simulink model "fullmodel"  (R2024b)
settings: Solver=VariableStepAuto  StartTime=0.0  StopTime=10.0  RelTol=1e-3
libraries: simulink x1
settings Model: Creator=ryandavis  LastModifiedBy=Cory

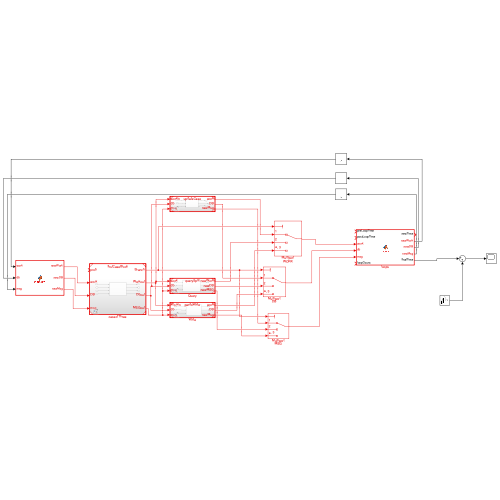
[thumbnail: Simulink's stored preview of the top-level diagram]
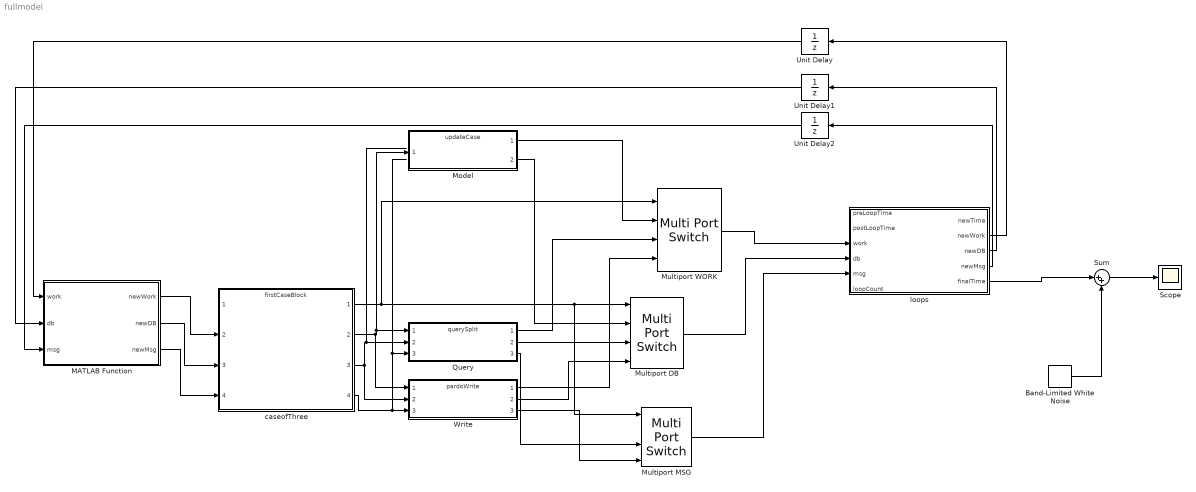
== system fullmodel ==
  Band-Limited White Noise : simulink/Sources/Band-Limited White Noise  Cov=[0.1]  Ts=0.1  seed=[23341]
  MATLAB Function : MATLAB Function  TreatAsAtomicUnit=on
  Model : ModelReference  ModelNameDialog=updateCase.slx  SimulationMode=Normal  ModelReferenceVersion=1.5
  Multiport DB : MultiPortSwitch  SaturateOnIntegerOverflow=off  InputSameDT=off
  Multiport MSG : MultiPortSwitch  SaturateOnIntegerOverflow=off  InputSameDT=off
  Multiport WORK : MultiPortSwitch  SaturateOnIntegerOverflow=off  InputSameDT=off
  Query : ModelReference  ModelNameDialog=querySplit.slx  SimulationMode=Normal  ModelReferenceVersion=1.7
  Scope : Scope
  Sum : Sum  Inputs=|++
  Unit Delay : UnitDelay  SampleTime=-1  HasFrameUpgradeWarning=on
  Unit Delay1 : UnitDelay  SampleTime=-1  HasFrameUpgradeWarning=on
  Unit Delay2 : UnitDelay  SampleTime=-1  HasFrameUpgradeWarning=on
  Write : ModelReference  ModelNameDialog=pardoWrite.slx  SimulationMode=Normal  ModelReferenceVersion=1.7
  caseofThree : ModelReference  ModelNameDialog=firstCaseBlock.slx  SimulationMode=Normal  ModelReferenceVersion=1.5
  loops : MATLAB Function  TreatAsAtomicUnit=on
  wires:
  MATLAB Function/3(newMsg) -> caseofThree/4
  MATLAB Function/2(newDB) -> caseofThree/3
  MATLAB Function/1(newWork) -> caseofThree/2
  caseofThree/1 -> Multiport WORK/1, Multiport MSG/1, Multiport DB/1
  Model/1 -> Multiport WORK/2
  Query/1 -> Multiport WORK/3
  Write/1 -> Multiport WORK/4
  Model/2 -> Multiport DB/2
  Query/2 -> Multiport DB/3
  ? -> Multiport MSG/2
  Write/2 -> Multiport DB/4
  Query/3 -> Multiport MSG/3
  Write/3 -> Multiport MSG/4
  Multiport WORK/1 -> loops/3(work)
  Multiport DB/1 -> loops/4(db)
  Multiport MSG/1 -> loops/5(msg)
  caseofThree/2 -> Write/1, Query/1, Model/1
  caseofThree/3 -> Write/2, Query/2
  caseofThree/4 -> Query/3, Write/3
  loops/5(finalTime) -> Sum/1
  Band-Limited White Noise/1 -> Sum/2
  Sum/1 -> Scope/1
  loops/2(newWork) -> Unit Delay/1
  loops/3(newDB) -> Unit Delay1/1
  loops/4(newMsg) -> Unit Delay2/1
  Unit Delay/1 -> MATLAB Function/1(work)
  Unit Delay1/1 -> MATLAB Function/2(db)
  Unit Delay2/1 -> MATLAB Function/3(msg)

== matlab function fullmodel/MATLAB Function ==
  data: work input; newWork output; db input; msg input; newDB output; newMsg output
function [newWork, newDB, newMsg] = initialize(work, db, msg)
    workIncrement = 2;
    dbIncrement = 1;
    msgIncrement = 1;
    
    newWork = work + workIncrement;
    newDB = db + dbIncrement;
    newMsg = msg + msgIncrement;
end

== matlab function fullmodel/loops ==
  data: preLoopTime input; postLoopTime input; newTime output; work input; db input; msg input; newWork output; newDB output; newMsg output; finalTime output; loopCount input
function [newTime, newWork, newDB, newMsg, finalTime] = Loop(preLoopTime, postLoopTime, work, db, msg, loopCount)
    newTime = preLoopTime + loopCount * (postLoopTime - preLoopTime);

    workIncrement = 10;
    dbIncrement = 20;
    msgIncrement = 5;
    
    newWork = work + loopCount * workIncrement;
    newDB = db + loopCount * dbIncrement;
    newMsg = msg + loopCount * msgIncrement;
    
    if loopCount == 2
        cpuQuantity = 3;
        diskQuantity = 2;
        networkQuantity = 1;

        cpuServiceTime = 0.0001;
        diskServiceTime = 0.02;
        networkServiceTime = 0.1;

        cpuTime = cpuQuantity * cpuServiceTime * newWork;
        diskTime = diskQuantity * diskServiceTime * newDB;
        networkTime = networkQuantity * networkServiceTime * newMsg;

        finalTime = cpuTime + diskTime + networkTime;
    else
        finalTime = 0;  
    end
end
